simulink library "powerlib"  (Simulink 6.0)
settings: Solver=ode45  SolverMode=SingleTasking  StartTime=0.0  StopTime=10.0  RelTol=1e-3
undefined symbols (not defined in the file or in its folder): com, ctrl1, Da, DiscIntNeverNeededParam, dtha, etat, FA, find_system, Ha, j, Ka, Ki, Kv, q0, Rground, sel, st_a, st_b, st_c, sta, stb, stc, T1, T2, T3, T4
libraries: powerlib_models x30, powerlib x25, simulink_extras x6, powerlib_extras x3, simulink x2
(part 6 of 7)

== system powerlib/Machines/Excitation System ==
  note: The simulink model of the Excitation system
      | can be found in the Continuous and Discrete
      | libraries of powerlib_models.
  vref : Inport  Port=1  LatchInput=off
  vd : Inport  Port=2  LatchInput=off
  vq : Inport  Port=3  LatchInput=off
  vstab : Inport  Port=4  LatchInput=off
  Source : powerlib_models/Continuous/Excitation_System  tr=tr  reg=reg  exc=exc  tgr=tgr  damp=damp  sat=sat  lim=lim  v0=v0
  Vf : Outport  InitialOutput=0
  wires:
  Source/1 -> Vf/1
  vref/1 -> Source/1
  vd/1 -> Source/2
  vq/1 -> Source/3
  vstab/1 -> Source/4

== system powerlib/Machines/Generic Power System Stabilizer ==
  note: The simulink model of the Generic Power
      | System Stabilizer can be found in the
      | Continuous and Discrete libraries
      | of powerlib_models.
  In : Inport  Port=1  LatchInput=off
  Source : powerlib_models/Continuous/PSS  Tsensor=Tsensor  K=K  Twashout=Twashout  Tleadlag1=Tleadlag1  Tleadlag2=Tleadlag2  VSlimits=VSlimits  Vinit=Vinit  Plot_On=off  MagdB_On=on  FreqRange=logspace(-2,2,500)
  Vstab : Outport  InitialOutput=0
  wires:
  Source/1 -> Vstab/1
  In/1 -> Source/1

== system powerlib/Machines/Hydraulic Turbine and Governor ==
  note: The simulink model of the Hydraulic Turbine and
      | Governor can be found in the Continuous and
      | Discrete libraries of powerlib_models.
  wref : Inport  Port=1  LatchInput=off
  Pref : Inport  Port=2  LatchInput=off
  we : Inport  Port=3  LatchInput=off
  Pe0 : Inport  Port=4  LatchInput=off
  dw : Inport  Port=5  LatchInput=off
  Source : powerlib_models/Continuous/HTG  sm=sm  gate=gate  reg=reg  hyd=hyd  dref=dref  po=po
  Pm : Outport  InitialOutput=0
  gate : Outport  Port=2  InitialOutput=0
  wires:
  wref/1 -> Source/1
  Pref/1 -> Source/2
  we/1 -> Source/3
  Pe0/1 -> Source/4
  dw/1 -> Source/5
  Source/2 -> gate/1
  Source/1 -> Pm/1

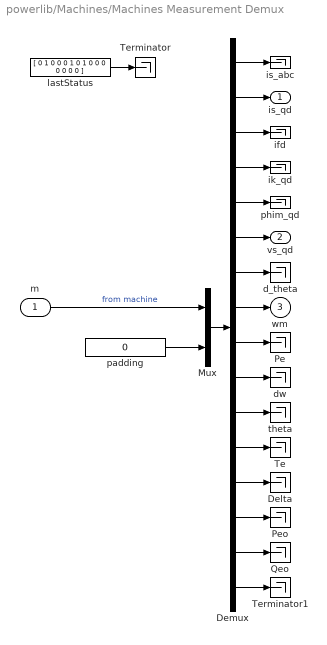
== system powerlib/Machines/Machines Measurement Demux ==
  m : Inport  Port=1  LatchInput=off
  Delta : Terminator
      settings: Tag=port13
  Demux : Demux  Outputs="[3 2 1 3 2 2 1 1 1 1 1 1 1 1 1,  1]"
  Mux : Mux  Inputs=2
  Pe : Terminator
      settings: Tag=port9
  Peo : Terminator
      settings: Tag=port14
  Qeo : Terminator
      settings: Tag=port15
  Te : Terminator
      settings: Tag=port12
  Terminator : Terminator
  Terminator1 : Terminator
  d_theta : Terminator
      settings: Tag=port7
  dw : Terminator
      settings: Tag=port10
  ifd : Terminator
      settings: Tag=port3
  ik_qd : Terminator
      settings: Tag=port4
  is_abc : Terminator
      settings: Tag=port1
  lastStatus : Constant  Value="[ 0  1  0  0  0  1  0  1  0  0  0  0  0  0  0 ]"
  padding : Constant  Value=0
  phim_qd : Terminator
      settings: Tag=port5
  theta : Terminator
      settings: Tag=port11
  is_qd : Outport  Tag=port2
  vs_qd : Outport  Tag=port6  Port=2
  wm : Outport  Tag=port8  Port=3
  wires:
  padding/1 -> Mux/2
  Demux/1 -> is_abc/1
  Demux/2 -> is_qd/1
  Demux/3 -> ifd/1
  Demux/4 -> ik_qd/1
  Demux/5 -> phim_qd/1
  Demux/6 -> vs_qd/1
  Demux/7 -> d_theta/1
  Demux/8 -> wm/1
  Demux/9 -> Pe/1
  Demux/10 -> dw/1
  Demux/11 -> theta/1
  Mux/1 -> Demux/1
  lastStatus/1 -> Terminator/1
  m/1 -> Mux/1  "from machine"
  Demux/16 -> Terminator1/1
  Demux/15 -> Qeo/1
  Demux/14 -> Peo/1
  Demux/13 -> Delta/1
  Demux/12 -> Te/1

== system powerlib/Machines/Multi-Band Power System Stabilizer ==
  note: The simulink model of the Multi-Band Power
      | System Stabilizer can be found in the
      | Continuous and Discrete libraries
      | of powerlib_models.
  dw : Inport  Port=1  LatchInput=off
  Source : powerlib_models/Continuous/MBPSS  OperationMode=Simplified settings  Kg=Kg  GL=GL  GI=GI  GH=GH  GLd=GLd  TcLF=TcLF  GId=GId  TcIF=TcIF  GHd=GHd  TcHF=TcHF  LIM=LIM  Plot_On=off  MagdB_On=off  FreqRange=logspace(-2,2,500)
  Vstab : Outport  InitialOutput=0
  wires:
  dw/1 -> Source/1
  Source/1 -> Vstab/1

== system powerlib/Machines/Permanent Magnet Synchronous Machine ==
  Tm : Inport  Orientation=left  Port=1  LatchInput=off
  ASM : PMComponent  PhysicalDomain=powersysdomain  LeftPortType=p1  RightPortType=p1  LConnTagsString=A|B  RConnTagsString=__newr0
      mask Type: InnerPowersysBlock
  Measurement list : Subsystem
  PMSM_mechanics : powerlib_models/Continuous/PMSM_mechanics  Orientation=left
  Source : powerlib_models/Continuous/PM_synchronous_machine
  A : PMIOPort  Port=1  Side=Left
  B : PMIOPort  Port=2  Side=Left
  C : PMIOPort  Orientation=left  Port=3  Side=Left
  m : Outport  InitialOutput=0
  tag scope: LibraryTag=global
  wires:
  Measurement list/1(Out1) -> m/1
  [LibraryTag] -> Source/1
  Source/1 -> [LibraryTag]
  Source/3 -> PMSM_mechanics/2
  Source/2 -> Measurement list/1(m_e)
  Tm/1 -> PMSM_mechanics/1
  PMSM_mechanics/3 -> Measurement list/2(m_m)
  PMSM_mechanics/2 -> Source/3
  PMSM_mechanics/1 -> Source/2
  connections:
  C/RConn1 -- ASM/RConn1
  B/RConn1 -- ASM/LConn2
  A/RConn1 -- ASM/LConn1

== system powerlib/Machines/Simplified Synchronous Machine SI Units ==
  Pm : Inport  Orientation=left  Port=1  LatchInput=off
  E : Inport  Port=2  LatchInput=off
  Measurement list : Subsystem
  SSM : PMComponent  PhysicalDomain=powersysdomain  LeftPortType=p1  RightPortType=p1  LConnTagsString=__newl0  RConnTagsString=A|B|C
      mask Type: InnerPowersysBlock
  SSM_mechanics : powerlib_models/Continuous/SSM_mechanics  Orientation=left
  Source : powerlib_models/Continuous/simplified_sync_mach
  A : PMIOPort  Orientation=left  Port=1  Side=Right
  B : PMIOPort  Orientation=left  Port=2  Side=Right
  C : PMIOPort  Orientation=left  Port=3  Side=Right
  m : Outport  InitialOutput=0
  tag scope: LibraryTag=global
  wires:
  Measurement list/1(Out1) -> m/1
  [LibraryTag] -> Source/1
  E/1 -> Source/2
  Source/1 -> [LibraryTag]
  Source/2 -> Measurement list/1(In1)
  Source/3 -> SSM_mechanics/2
  Pm/1 -> SSM_mechanics/1
  SSM_mechanics/1 -> Source/3
  SSM_mechanics/2 -> Source/4
  connections:
  SSM/RConn3 -- C/RConn1
  SSM/RConn1 -- A/RConn1
  SSM/RConn2 -- B/RConn1

== system powerlib/Machines/Simplified Synchronous Machine pu Units ==
  Pm : Inport  Orientation=left  Port=1  LatchInput=off
  E : Inport  Port=2  LatchInput=off
  Measurement list : Subsystem
  SSM : PMComponent  PhysicalDomain=powersysdomain  LeftPortType=p1  RightPortType=p1  LConnTagsString=__newl0  RConnTagsString=A|B|C
      mask Type: InnerPowersysBlock
  SSM_mechanics : powerlib_models/Continuous/SSM_mechanics  Orientation=left
  Source : powerlib_models/Continuous/simplified_sync_mach
  A : PMIOPort  Orientation=left  Port=1  Side=Right
  B : PMIOPort  Orientation=left  Port=2  Side=Right
  C : PMIOPort  Orientation=left  Port=3  Side=Right
  m : Outport  InitialOutput=0
  tag scope: LibraryTag=global
  wires:
  Measurement list/1(Out1) -> m/1
  [LibraryTag] -> Source/1
  Source/1 -> [LibraryTag]
  Source/2 -> Measurement list/1(In1)
  Pm/1 -> SSM_mechanics/1
  Source/3 -> SSM_mechanics/2
  E/1 -> Source/2
  SSM_mechanics/1 -> Source/3
  SSM_mechanics/2 -> Source/4
  connections:
  SSM/RConn3 -- C/RConn1
  SSM/RConn1 -- A/RConn1
  SSM/RConn2 -- B/RConn1

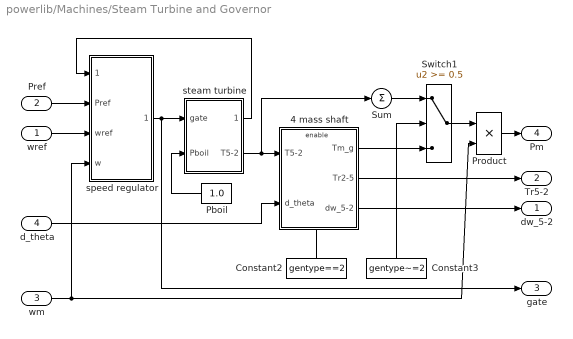
== system powerlib/Machines/Steam Turbine and Governor ==
  wref : Inport  Port=1  LatchInput=off
  Pref : Inport  Port=2  LatchInput=off
  wm : Inport  Port=3  LatchInput=off
  d_theta : Inport  Port=4  LatchInput=off
  4 mass shaft : Subsystem  TreatAsAtomicUnit=on
  Constant2 : Constant  Orientation=up  Value=gentype==2
  Constant3 : Constant  Orientation=up  Value=gentype~=2
  Pboil : Constant  Orientation=left  Value=1.0
  Product : Product  SaturateOnIntegerOverflow=on  InputSameDT=on
  Sum : Sum  Inputs=+  SaturateOnIntegerOverflow=on  InputSameDT=on
  Switch1 : Switch  Threshold=0.5  InputSameDT=on
  speed regulator : Subsystem  mask(Speed regulator for thermal turbine){Rp=reg1(2), Kp=reg1(1), Dz=reg1(3), Tsr=reg2(1), Tsm=reg2(2), lim=reg3, g0=q0}
      mask prompts: Rp "Permanent droop Rp:"; Kp "Regulator gain Kp:"; Dz "Regulator dead zone limit Dz (p.u.):"; Tsr "Speed relay time constant Tsr (s):"; Tsm "Servo motor time constant Tsv:"; lim "Gate opening limits [ vgmin,vgmax (p.u./s)  gmin,gmax (p.u.)]:"; g0 "Initial gate opening g0 (p.u.):"
      mask init:
      | vgmin=lim(1); vgmax=lim(2); gmin=lim(3); gmax=lim(4);
  steam turbine : Subsystem  mask(Thermal turbine){Fa=FA, Ta=turb1, f0=q0}
      mask prompts: Fa "Generator 1 torque fractions [ F1  F2  F3  F4 ]:"; Ta "Time constants [ T1  T2  T3  T4 ] (s):"; f0 "Initial flows f0:"
      mask init:
      | F2=Fa(1); F3=Fa(2); F4=Fa(3); F5=Fa(4);
      | if Ta(1)==0, T1=1; else T1=Ta(1); end; if Ta(2)==0, T2=1; else T2=Ta(2); end
      | if Ta(3)==0, T3=1; else T3=Ta(3); end; if Ta(4)==0, T4=1; else T4=Ta(4); end
  dw_5-2 : Outport
  Tr5-2 : Outport  Port=2
  gate : Outport  Port=3
  Pm : Outport  Port=4
  wires:
  wm/1 -> Product/2, speed regulator/4(w)
  Pref/1 -> speed regulator/2(Pref)
  wref/1 -> speed regulator/3(wref)
  Pboil/1 -> steam turbine/2(Pboil)
  Product/1 -> Pm/1
  4 mass shaft/2(Tr2-5) -> Tr5-2/1
  Switch1/1 -> Product/1
  4 mass shaft/1(Tm_g) -> Switch1/3
  Sum/1 -> Switch1/1
  Constant3/1 -> Switch1/2
  d_theta/1 -> 4 mass shaft/2(d_theta)
  steam turbine/1(flowHp) -> speed regulator/1(flowHP)
  steam turbine/2(T5-2) -> 4 mass shaft/1(T5-2), Sum/1
  4 mass shaft/3(dw_5-2) -> dw_5-2/1
  speed regulator/1(gate opening) -> steam turbine/1(gate), gate/1
  Constant2/1 -> 4 mass shaft/Enable

== system powerlib/Machines/Synchronous Machine SI Fundamental ==
  Pm : Inport  Orientation=left  Port=1  LatchInput=off
  Vf_ : Inport  Port=2  LatchInput=off
  Measurement list : Subsystem
  SM : PMComponent  PhysicalDomain=powersysdomain  LeftPortType=p1  RightPortType=p1  LConnTagsString=__newl0  RConnTagsString=B|C
      mask Type: InnerPowersysBlock
  SM_mechanics : powerlib_models/Continuous/SM_mechanics  Orientation=left
  Source : powerlib_models/Continuous/synchronous_machine
  A : PMIOPort  Port=1  Side=Right
  B : PMIOPort  Orientation=left  Port=2  Side=Right
  C : PMIOPort  Orientation=left  Port=3  Side=Right
  m : Outport  InitialOutput=0
  tag scope: LibraryTag=global
  wires:
  Source/1 -> [LibraryTag]
  [LibraryTag] -> Source/1
  Source/3 -> SM_mechanics/1
  Vf_/1 -> Source/2
  Measurement list/1(m) -> m/1
  SM_mechanics/1 -> Measurement list/2(m_m)
  Source/2 -> Measurement list/1(m_e)
  SM_mechanics/2 -> Source/3
  SM_mechanics/3 -> Source/4
  Pm/1 -> SM_mechanics/2
  connections:
  SM/RConn2 -- C/RConn1
  SM/LConn1 -- A/RConn1
  SM/RConn1 -- B/RConn1

== system powerlib/Machines/Synchronous Machine pu Fundamental ==
  Pm : Inport  Orientation=left  Port=1  LatchInput=off
  Vf_ : Inport  Port=2  LatchInput=off
  Measurement list : Subsystem
  SM : PMComponent  PhysicalDomain=powersysdomain  LeftPortType=p1  RightPortType=p1  LConnTagsString=__newl0  RConnTagsString=B|C
      mask Type: InnerPowersysBlock
  SM_mechanics : powerlib_models/Continuous/SM_mechanics  Orientation=left
  Source : powerlib_models/Continuous/synchronous_machine
  A : PMIOPort  Port=1  Side=Right
  B : PMIOPort  Orientation=left  Port=2  Side=Right
  C : PMIOPort  Orientation=left  Port=3  Side=Right
  m : Outport  InitialOutput=0
  tag scope: LibraryTag=global
  wires:
  Measurement list/1(m) -> m/1
  Source/1 -> [LibraryTag]
  [LibraryTag] -> Source/1
  Vf_/1 -> Source/2
  Pm/1 -> SM_mechanics/2
  Source/3 -> SM_mechanics/1
  Source/2 -> Measurement list/1(m_e)
  SM_mechanics/1 -> Measurement list/2(m_m)
  SM_mechanics/2 -> Source/3
  SM_mechanics/3 -> Source/4
  connections:
  C/RConn1 -- SM/RConn2
  B/RConn1 -- SM/RConn1
  A/RConn1 -- SM/LConn1

== system powerlib/Machines/Synchronous Machine pu Standard ==
  Pm : Inport  Orientation=left  Port=1  LatchInput=off
  Vf_ : Inport  Port=2  LatchInput=off
  Measurement list : Subsystem
  SM : PMComponent  PhysicalDomain=powersysdomain  LeftPortType=p1  RightPortType=p1  LConnTagsString=__newl0  RConnTagsString=B|C
      mask Type: InnerPowersysBlock
  SM_mechanics : powerlib_models/Continuous/SM_mechanics  Orientation=left
  Source : powerlib_models/Continuous/synchronous_machine
  A : PMIOPort  Port=1  Side=Right
  B : PMIOPort  Orientation=left  Port=2  Side=Right
  C : PMIOPort  Orientation=left  Port=3  Side=Right
  m : Outport  InitialOutput=0
  tag scope: LibraryTag=global
  wires:
  Source/1 -> [LibraryTag]
  [LibraryTag] -> Source/1
  Source/3 -> SM_mechanics/1
  Vf_/1 -> Source/2
  Source/2 -> Measurement list/1(m_e)
  SM_mechanics/1 -> Measurement list/2(m_m)
  Measurement list/1(m) -> m/1
  SM_mechanics/2 -> Source/3
  SM_mechanics/3 -> Source/4
  Pm/1 -> SM_mechanics/2
  connections:
  A/RConn1 -- SM/LConn1
  SM/RConn2 -- C/RConn1
  SM/RConn1 -- B/RConn1

== system powerlib/Measurements/  Extra Library  ==

== system powerlib/Measurements/  Extra Library 1 ==

== system powerlib/Measurements/  Extra Library 2 ==

== system powerlib/Measurements/Current Measurement ==
  CurrentMeasurement : PMComponent  PhysicalDomain=powersysdomain  LeftPortType=p1  RightPortType=p1  LConnTagsString=a  RConnTagsString=__new0
      mask Type: InnerPowersysBlock
  model : powerlib_models/Continuous/Measurement
  + : PMIOPort  Port=1  Side=Left
  - : PMIOPort  Orientation=left  Port=2  Side=Right
  i : Outport  InitialOutput=0
  wires:
  [LibraryTag] -> model/1
  model/1 -> i/1
  connections:
  -/RConn1 -- CurrentMeasurement/RConn1
  +/RConn1 -- CurrentMeasurement/LConn1

== system powerlib/Measurements/Multimeter ==
  Gain2 : Gain  Gain=Gain  SaturateOnIntegerOverflow=on
  Mode : Constant  Value=Display
  Selector : Selector  Elements=SelectionMode  InputPortWidth=SignalLength
  StoreData : Subsystem  Orientation=down  TreatAsAtomicUnit=on  mask{RowMax=inf}
      mask prompts: RowMax "Maximum Number of rows"
      mask init:
      | powericon('psbloadfunction',gcb,'StoreDataBlock','Initialize');
      settings: CopyFcn=powericon('psbloadfunction',gcb,'StoreDataBlock','UpdateVariableName');
  model : powerlib_models/Continuous/Measurement
  selection : Selector  Elements=sel  InputPortWidth=L
  Out1 : Outport
  wires:
  Mode/1 -> StoreData/Enable
  selection/1 -> Gain2/1
  [gotomultimeterPSB] -> selection/1
  Gain2/1 -> model/1
  model/1 -> Selector/1
  Selector/1 -> Out1/1, StoreData/1(In1)

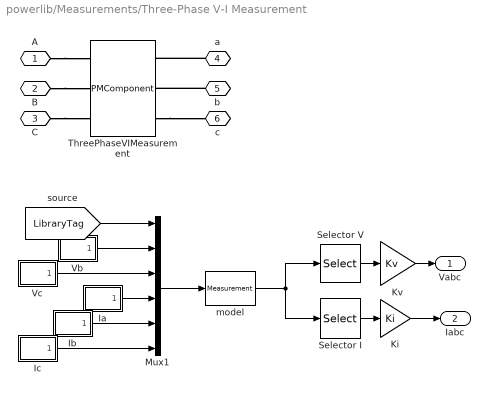
== system powerlib/Measurements/Three-Phase V-I Measurement ==
  Ia : Subsystem
  Ib : Subsystem
  Ic : Subsystem
  Ki : Gain  Gain=Ki  SaturateOnIntegerOverflow=on
  Kv : Gain  Gain=Kv  SaturateOnIntegerOverflow=on
  Mux1 : Mux  Inputs=6
  Selector I : Selector  Elements=SelectionModeI  InputPortWidth=SignalLength
  Selector V : Selector  Elements=SelectionModeV  InputPortWidth=SignalLength
  ThreePhaseVIMeasurement : PMComponent  PhysicalDomain=powersysdomain  LeftPortType=p1  RightPortType=p1  LConnTagsString=A|B|C  RConnTagsString=a|b|c
      mask Type: InnerPowersysBlock
  Vb : Subsystem
  Vc : Subsystem
  model : powerlib_models/Continuous/Measurement
  A : PMIOPort  Port=1  Side=Left
  B : PMIOPort  Port=2  Side=Left
  C : PMIOPort  Port=3  Side=Left
  a : PMIOPort  Orientation=left  Port=4  Side=Right
  b : PMIOPort  Orientation=left  Port=5  Side=Right
  c : PMIOPort  Orientation=left  Port=6  Side=Right
  Vabc : Outport
  Iabc : Outport  Port=2
  wires:
  Vb/1(Out1) -> Mux1/2
  Vc/1(Out1) -> Mux1/3
  Ia/1(Out1) -> Mux1/4
  Ib/1(Out1) -> Mux1/5
  Ic/1(Out1) -> Mux1/6
  [LibraryTag] -> Mux1/1
  Selector I/1 -> Ki/1
  Selector V/1 -> Kv/1
  Ki/1 -> Iabc/1
  Kv/1 -> Vabc/1
  Mux1/1 -> model/1
  model/1 -> Selector V/1, Selector I/1
  connections:
  B/RConn1 -- ThreePhaseVIMeasurement/LConn2
  A/RConn1 -- ThreePhaseVIMeasurement/LConn1
  C/RConn1 -- ThreePhaseVIMeasurement/LConn3
  ThreePhaseVIMeasurement/RConn3 -- c/RConn1
  b/RConn1 -- ThreePhaseVIMeasurement/RConn2
  a/RConn1 -- ThreePhaseVIMeasurement/RConn1

== system powerlib/Measurements/Voltage Measurement ==
  VoltageMeasurement : PMComponent  PhysicalDomain=powersysdomain  LeftPortType=p1  RightPortType=p1  LConnTagsString=+  RConnTagsString=-
      mask Type: InnerPowersysBlock
  model : powerlib_models/Continuous/Measurement
  + : PMIOPort  Port=1  Side=Left
  - : PMIOPort  Orientation=left  Port=2  Side=Left
  v : Outport  InitialOutput=0
  wires:
  [LibraryTag] -> model/1
  model/1 -> v/1
  connections:
  +/RConn1 -- VoltageMeasurement/LConn1
  -/RConn1 -- VoltageMeasurement/RConn1

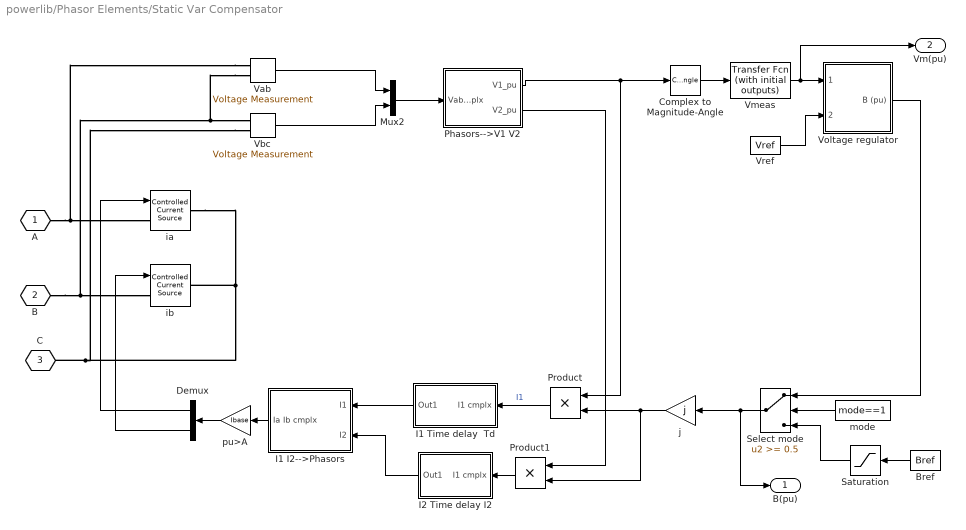
== system powerlib/Phasor Elements/Static Var Compensator ==
  Bref : Constant  Orientation=left  Value=Bref
  Complex to Magnitude-Angle : ComplexToMagnitudeAngle  Output=Magnitude
  Demux : Demux  Orientation=left  Outputs=2
  I1 I2-->Phasors : Subsystem  Orientation=left
  I1 Time delay  Td : Subsystem  Orientation=left
  I2 Time delay I2 : Subsystem  Orientation=left
  Mux2 : Mux  Inputs=2
  Phasors-->V1 V2 : Subsystem
  Product : Product  Orientation=left  SaturateOnIntegerOverflow=on  InputSameDT=on
  Product1 : Product  Orientation=left  SaturateOnIntegerOverflow=on  InputSameDT=on
  Saturation : Saturate  Orientation=left  UpperLimit=Bmax  LowerLimit=Bmin
  Select mode : Switch  Orientation=left  Threshold=0.5  InputSameDT=on
  Vab : powerlib/Measurements/Voltage Measurement  PhasorSimulation=off  OutputType=Complex  PSBequivalent=0
  Vbc : powerlib/Measurements/Voltage Measurement  PhasorSimulation=off  OutputType=Complex  PSBequivalent=0
  Vmeas : simulink_extras/Additional Linear/Transfer Fcn (with initial outputs)  N=[1]  D="[Tm  1]"  Y0=Vref  U0=Vref
  Voltage regulator : Subsystem
  Vref : Constant  Value=Vref
  ia : powerlib/Electrical Sources/Controlled Current Source  Description=source block  Initialize=off  Amplitude=0  Phase=0  Frequency=0  Measurements=None
  ib : powerlib/Electrical Sources/Controlled Current Source  Description=source block  Initialize=off  Amplitude=0  Phase=0  Frequency=0  Measurements=None
  j : Gain  Orientation=left  Gain=j  SaturateOnIntegerOverflow=on
  mode : Constant  Orientation=left  Value=mode==1
  pu>A : Gain  Orientation=left  Gain=Ibase  SaturateOnIntegerOverflow=on
  A : PMIOPort  Port=1  Side=Left
  B : PMIOPort  Port=2  Side=Left
  C : PMIOPort  Port=3  Side=Left
  B(pu) : Outport
  Vm(pu) : Outport  Port=2
  wires:
  Saturation/1 -> Select mode/3
  Demux/2 -> ib/1
  Demux/1 -> ia/1
  mode/1 -> Select mode/2
  Voltage regulator/1(B (pu)) -> Select mode/1
  Bref/1 -> Saturation/1
  Select mode/1 -> B(pu)/1, j/1
  Mux2/1 -> Phasors-->V1 V2/1(Vab Vbc cmplx)
  Phasors-->V1 V2/1(V1_pu) -> Complex to Magnitude-Angle/1, Product/1
  Vref/1 -> Voltage regulator/2(Vref (pu))
  Vmeas/1 -> Voltage regulator/1(V1meas (pu)), Vm(pu)/1
  I1 I2-->Phasors/1(Ia Ib cmplx) -> pu>A/1
  I2 Time delay I2/1(Out1) -> I1 I2-->Phasors/2(I2)
  Complex to Magnitude-Angle/1 -> Vmeas/1
  Vab/1 -> Mux2/1
  Vbc/1 -> Mux2/2
  I1 Time delay  Td/1(Out1) -> I1 I2-->Phasors/1(I1)
  pu>A/1 -> Demux/1
  Product/1 -> I1 Time delay  Td/1(I1 cmplx)  "I1"
  j/1 -> Product/2, Product1/2
  Phasors-->V1 V2/2(V2_pu) -> Product1/1
  Product1/1 -> I2 Time delay I2/1(I1 cmplx)
  connections:
  Vbc/LConn2 -- C/RConn1 -- ib/RConn1 -- ia/RConn1
  Vab/LConn2 -- Vbc/LConn1 -- ib/LConn1 -- B/RConn1
  Vab/LConn1 -- ia/LConn1 -- A/RConn1

== system powerlib/Power Electronics/  Extra Library  ==

== system powerlib/Power Electronics/  Extra Library 1 ==

== system powerlib/Power Electronics/Detailed Thyristor ==
  g : Inport  Port=1  LatchInput=off
  DetailedThyristor : PMComponent  PhysicalDomain=powersysdomain  LeftPortType=p1  RightPortType=p1  LConnTagsString=a  RConnTagsString=__new0
      mask Type: InnerPowersysBlock
  Measurement list : Subsystem
  a : PMIOPort  Port=1  Side=Left
  k : PMIOPort  Orientation=left  Port=2  Side=Right
  m : Outport  InitialOutput=0
  tag scope: LibraryTag=global
  wires:
  g/1 -> [LibraryTag]
  [LibraryTag] -> Measurement list/1(In1)
  Measurement list/1(Out1) -> m/1
  connections:
  DetailedThyristor/RConn1 -- k/RConn1
  a/RConn1 -- DetailedThyristor/LConn1

== system powerlib/Power Electronics/Diode ==
  Diode : PMComponent  PhysicalDomain=powersysdomain  LeftPortType=p1  RightPortType=p1  LConnTagsString=a  RConnTagsString=__new0
      mask Type: InnerPowersysBlock
  Measurement list : Subsystem
  m : Terminator
  a : PMIOPort  Port=1  Side=Left
  k : PMIOPort  Orientation=left  Port=2  Side=Right
  wires:
  [LibraryTag] -> Measurement list/1(In1)
  Measurement list/1(Out1) -> m/1
  connections:
  Diode/RConn1 -- k/RConn1
  a/RConn1 -- Diode/LConn1

== system powerlib/Power Electronics/Gto ==
  g : Inport  Port=1  LatchInput=off
  GTO : PMComponent  PhysicalDomain=powersysdomain  LeftPortType=p1  RightPortType=p1  LConnTagsString=a  RConnTagsString=__new0
      mask Type: InnerPowersysBlock
  Measurement list : Subsystem
  a : PMIOPort  Port=1  Side=Left
  k : PMIOPort  Orientation=left  Port=2  Side=Right
  m : Outport  InitialOutput=0
  tag scope: LibraryTag=global
  wires:
  g/1 -> [LibraryTag]
  [LibraryTag] -> Measurement list/1(In1)
  Measurement list/1(Out1) -> m/1
  connections:
  GTO/RConn1 -- k/RConn1
  a/RConn1 -- GTO/LConn1

== system powerlib/Power Electronics/IGBT ==
  g : Inport  Port=1  LatchInput=off
  IGBT : PMComponent  PhysicalDomain=powersysdomain  LeftPortType=p1  RightPortType=p1  LConnTagsString=a  RConnTagsString=__new0
      mask Type: InnerPowersysBlock
  Measurement list : Subsystem
  C : PMIOPort  Port=1  Side=Left
  E : PMIOPort  Orientation=left  Port=2  Side=Right
  m : Outport
  tag scope: LibraryTag=global
  wires:
  [LibraryTag] -> Measurement list/1(In1)
  g/1 -> [LibraryTag]
  Measurement list/1(Out1) -> m/1
  connections:
  IGBT/RConn1 -- E/RConn1
  C/RConn1 -- IGBT/LConn1

== system powerlib/Power Electronics/Ideal Switch ==
  g : Inport  Port=1  LatchInput=off
  IdealSwitch : PMComponent  PhysicalDomain=powersysdomain  LeftPortType=p1  RightPortType=p1  LConnTagsString=a  RConnTagsString=__new0
      mask Type: InnerPowersysBlock
  Measurement list : Subsystem
  1 : PMIOPort  Port=1  Side=Left
  2 : PMIOPort  Orientation=left  Port=2  Side=Right
  m : Outport
  tag scope: LibraryTag=global
  wires:
  [LibraryTag] -> Measurement list/1(In1)
  g/1 -> [LibraryTag]
  Measurement list/1(Out1) -> m/1
  connections:
  IdealSwitch/RConn1 -- 2/RConn1
  1/RConn1 -- IdealSwitch/LConn1

== system powerlib/Power Electronics/Mosfet ==
  g : Inport  Port=1  LatchInput=off
  Measurement list : Subsystem
  Mosfet : PMComponent  PhysicalDomain=powersysdomain  LeftPortType=p1  RightPortType=p1  LConnTagsString=a  RConnTagsString=__new0
      mask Type: InnerPowersysBlock
  d : PMIOPort  Port=1  Side=Left
  s : PMIOPort  Orientation=left  Port=2  Side=Right
  m : Outport
  tag scope: LibraryTag=global
  wires:
  g/1 -> [LibraryTag]
  [LibraryTag] -> Measurement list/1(In1)
  Measurement list/1(Out1) -> m/1
  connections:
  Mosfet/RConn1 -- s/RConn1
  d/RConn1 -- Mosfet/LConn1

== system powerlib/Power Electronics/Three-Level Bridge ==
  g : Inport  Port=1  PortDimensions=4*Arms  LatchInput=off
  Logical Operator : Logic  OutDataTypeMode=Specify via dialog  LogicDataType=float('double')
  UniversalBridge : PMComponent  PhysicalDomain=powersysdomain  LeftPortType=p1  RightPortType=p1  LConnTagsString=A|B|C  RConnTagsString=+|N|-
      mask Type: InnerPowersysBlock
  s1 : Selector  Elements=selection1  InputPortWidth=4*Arms
  s2 : Selector  Elements=selection2  InputPortWidth=4*Arms
  A : PMIOPort  Port=1  Side=Left
  B : PMIOPort  Port=2  Side=Left
  C : PMIOPort  Port=3  Side=Left
  + : PMIOPort  Orientation=left  Port=4  Side=Right
  N : PMIOPort  Orientation=left  Port=5  Side=Right
  - : PMIOPort  Orientation=left  Port=6  Side=Right
  tag scope: LibraryTag=global
  wires:
  g/1 -> s2/1, s1/1
  s2/1 -> Logical Operator/2
  s1/1 -> Logical Operator/1
  Logical Operator/1 -> [LibraryTag]
  connections:
  -/RConn1 -- UniversalBridge/RConn3
  UniversalBridge/RConn2 -- N/RConn1
  A/RConn1 -- UniversalBridge/LConn1
  B/RConn1 -- UniversalBridge/LConn2
  C/RConn1 -- UniversalBridge/LConn3
  UniversalBridge/RConn1 -- +/RConn1

== system powerlib/Power Electronics/Thyristor ==
  g : Inport  Port=1  LatchInput=off
  Measurement list : Subsystem
  Thyristor : PMComponent  PhysicalDomain=powersysdomain  LeftPortType=p1  RightPortType=p1  LConnTagsString=a  RConnTagsString=__new0
      mask Type: InnerPowersysBlock
  a : PMIOPort  Port=1  Side=Left
  k : PMIOPort  Orientation=left  Port=2  Side=Right
  m : Outport  InitialOutput=0
  tag scope: LibraryTag=global
  wires:
  g/1 -> [LibraryTag]
  [LibraryTag] -> Measurement list/1(In1)
  Measurement list/1(Out1) -> m/1
  connections:
  Thyristor/RConn1 -- k/RConn1
  a/RConn1 -- Thyristor/LConn1

== system powerlib/Power Electronics/Universal Bridge ==
  g : Inport  Port=1  LatchInput=off
  UniversalBridge : PMComponent  PhysicalDomain=powersysdomain  LeftPortType=p1  RightPortType=p1  LConnTagsString=A|B|C  RConnTagsString=+|-
      mask Type: InnerPowersysBlock
  A : PMIOPort  Port=1  Side=Left
  B : PMIOPort  Port=2  Side=Left
  C : PMIOPort  Port=3  Side=Left
  + : PMIOPort  Orientation=left  Port=4  Side=Right
  - : PMIOPort  Orientation=left  Port=5  Side=Right
  tag scope: LibraryTag=global
  wires:
  g/1 -> [LibraryTag]
  connections:
  UniversalBridge/RConn2 -- -/RConn1
  UniversalBridge/RConn1 -- +/RConn1
  A/RConn1 -- UniversalBridge/LConn1
  UniversalBridge/LConn2 -- B/RConn1
  UniversalBridge/LConn3 -- C/RConn1

== system powerlib/powergui/Subsystem ==

== system powerlib/Elements/Three-Phase Dynamic Load/Measurement list ==
  In1 : Inport  Port=1  LatchInput=off
  Bus Creator1 : BusCreator  DialogController=Simulink.DDGSource_Bus  Inputs=3
  Demux : Demux  Outputs=[1,1,1]
  Out1 : Outport
  wires:
  In1/1 -> Demux/1
  Bus Creator1/1 -> Out1/1
  Demux/2 -> Bus Creator1/2  "Active power P (W)"
  Demux/1 -> Bus Creator1/1  "Positive-sequence voltage V (pu)"
  Demux/3 -> Bus Creator1/3  "Reactive power Q (var)"

== system powerlib/Machines/Asynchronous Machine SI Units/Measurement list ==
  m_e : Inport  Port=1  LatchInput=off
  m_m : Inport  Port=2  LatchInput=off
  Bus Creator1 : BusCreator  DialogController=Simulink.DDGSource_Bus  Inputs=3
  Bus Creator2 : BusCreator  DialogController=Simulink.DDGSource_Bus  Inputs=9
  Bus Creator3 : BusCreator  DialogController=Simulink.DDGSource_Bus  Inputs=3
  Bus Creator4 : BusCreator  DialogController=Simulink.DDGSource_Bus  Inputs=9
  Demux : Demux  Outputs=[1,1,1,1,1,1,1,1,1,1,1,1,1,1,1,1,1,1]
  Demux1 : Demux  Outputs=[1,1,1]
  Out1 : Outport
  wires:
  Bus Creator3/1 -> Bus Creator1/3  "Mechanical"
  Demux/18 -> Bus Creator4/9  "Stator voltage vs_d (V)"
  Demux/17 -> Bus Creator4/8  "Stator voltage vs_q (V)"
  Demux/16 -> Bus Creator4/7  "Stator flux phis_d (V s)"
  Demux/15 -> Bus Creator4/6  "Stator flux phis_q (V s)"
  Demux1/1 -> Bus Creator3/1  "Rotor speed (wm)"
  Demux1/2 -> Bus Creator3/2  "Electromagnetic torque Te (N*m)"
  Demux1/3 -> Bus Creator3/3  "Rotor angle thetam (rad)"
  Bus Creator4/1 -> Bus Creator1/2  "Stator measurements"
  Demux/14 -> Bus Creator4/5  "Stator current is_d (A)"
  Demux/13 -> Bus Creator4/4  "Stator current  is_q (A)"
  Demux/12 -> Bus Creator4/3  "Stator current is_c (A)"
  Demux/11 -> Bus Creator4/2  "Stator current is_b (A)"
  Demux/10 -> Bus Creator4/1  "Stator current is_a (A)"
  Demux/9 -> Bus Creator2/9  "Rotor voltage Vr_d (V)"
  Demux/8 -> Bus Creator2/8  "Rotor voltage Vr_q (V)"
  Demux/7 -> Bus Creator2/7  "Rotor flux phir_d (V s)"
  Demux/6 -> Bus Creator2/6  "Rotor flux phir_q (V s)"
  Demux/5 -> Bus Creator2/5  "Rotor current  id (A)"
  Demux/4 -> Bus Creator2/4  "Rotor current  iq (A)"
  Bus Creator2/1 -> Bus Creator1/1  "Rotor measurements"
  Demux/3 -> Bus Creator2/3  "Rotor current ir_c (A)"
  Demux/2 -> Bus Creator2/2  "Rotor current ir_b (A)"
  Demux/1 -> Bus Creator2/1  "Rotor current ir_a (A)"
  Bus Creator1/1 -> Out1/1
  m_e/1 -> Demux/1
  m_m/1 -> Demux1/1

== system powerlib/Machines/Asynchronous Machine pu Units/Measurement list ==
  m_e : Inport  Port=1  LatchInput=off
  m_m : Inport  Port=2  LatchInput=off
  Bus Creator1 : BusCreator  DialogController=Simulink.DDGSource_Bus  Inputs=3
  Bus Creator2 : BusCreator  DialogController=Simulink.DDGSource_Bus  Inputs=9
  Bus Creator3 : BusCreator  DialogController=Simulink.DDGSource_Bus  Inputs=3
  Bus Creator4 : BusCreator  DialogController=Simulink.DDGSource_Bus  Inputs=9
  Demux : Demux  Outputs=[1,1,1,1,1,1,1,1,1,1,1,1,1,1,1,1,1,1]
  Demux1 : Demux  Outputs=[1,1,1]
  Out1 : Outport
  wires:
  m_e/1 -> Demux/1
  Bus Creator1/1 -> Out1/1
  Demux/1 -> Bus Creator2/1  "Rotor current ir_a (pu)"
  Demux/2 -> Bus Creator2/2  "Rotor current ir_b (pu)"
  Demux/3 -> Bus Creator2/3  "Rotor current ir_c (pu)"
  Bus Creator2/1 -> Bus Creator1/1  "Rotor measurements"
  Demux/4 -> Bus Creator2/4  "Rotor current  iq (pu)"
  Demux/5 -> Bus Creator2/5  "Rotor current  id (pu)"
  Demux/6 -> Bus Creator2/6  "Rotor flux phir_q (pu)"
  Demux/7 -> Bus Creator2/7  "Rotor flux phir_d (pu)"
  Demux/8 -> Bus Creator2/8  "Rotor voltage Vr_q (pu)"
  Demux/9 -> Bus Creator2/9  "Rotor voltage Vr_d (pu)"
  Demux/10 -> Bus Creator4/1  "Stator current is_a (pu)"
  Demux/11 -> Bus Creator4/2  "Stator current is_b (pu)"
  Demux/12 -> Bus Creator4/3  "Stator current is_c (pu)"
  Demux/13 -> Bus Creator4/4  "Stator current is_q (pu)"
  Demux/14 -> Bus Creator4/5  "Stator current is_d (pu)"
  Bus Creator4/1 -> Bus Creator1/2  "Stator measurements"
  Demux/15 -> Bus Creator4/6  "Stator flux phis_q (pu)"
  Demux/16 -> Bus Creator4/7  "Stator flux phis_d (pu)"
  Demux/17 -> Bus Creator4/8  "Stator voltage vs_q (pu)"
  Demux/18 -> Bus Creator4/9  "Stator voltage vs_d (pu)"
  Bus Creator3/1 -> Bus Creator1/3  "Mechanical"
  Demux1/1 -> Bus Creator3/1  "Rotor speed (wm)"
  Demux1/2 -> Bus Creator3/2  "Electromagnetic torque Te (pu)"
  Demux1/3 -> Bus Creator3/3  "Rotor angle thetam (rad)"
  m_m/1 -> Demux1/1

== system powerlib/Machines/DC Machine/Measurement list ==
  In1 : Inport  Port=1  LatchInput=off
  Bus Creator1 : BusCreator  DialogController=Simulink.DDGSource_Bus
  Demux : Demux  Outputs=[1,1,1,1]
  Out1 : Outport
  wires:
  In1/1 -> Demux/1
  Bus Creator1/1 -> Out1/1
  Demux/1 -> Bus Creator1/1  "Speed wm (rad/s)"
  Demux/2 -> Bus Creator1/2  "Armature current ia (A)"
  Demux/3 -> Bus Creator1/3  "Field current if (A)"
  Demux/4 -> Bus Creator1/4  "Electrical torque Te (n m)"

== system powerlib/Machines/DC Machine/Mechanics ==
  TL : Inport  Port=1  LatchInput=off
  ia : Inport  Port=2  LatchInput=off
  if : Inport  Port=3  LatchInput=off
  Coulomb (Tf) & Viscous ( Bm*w)  Friction Torques : simulink/Discontinuities/Coulomb & Viscous Friction  Orientation=left  offset=Tf  gain=Bm
  Gain2 : Gain  Gain=1/J  SaturateOnIntegerOverflow=on
  Integrator : Integrator  InitialCondition=w0  ZeroCross=off
  Mux : Mux
  Product : Product  SaturateOnIntegerOverflow=on  InputSameDT=on
  Product1 : Product  SaturateOnIntegerOverflow=on  InputSameDT=on
  Sum : Sum  Inputs=-+-  SaturateOnIntegerOverflow=on  InputSameDT=on
  Transfer Fcn2 : TransferFcn  Numerator=[Laf]  Denominator=[20e-6 1]
  FCEM : Outport
  m : Outport  Port=2
  wires:
  Coulomb (Tf) & Viscous ( Bm*w)  Friction Torques/1 -> Sum/3
  Transfer Fcn2/1 -> Product/2, Product1/2
  Product1/1 -> Mux/4, Sum/2  "Te"
  Integrator/1 -> Product/1, Mux/1, Coulomb (Tf) & Viscous ( Bm*w)  Friction Torques/1  "w"
  Gain2/1 -> Integrator/1
  Sum/1 -> Gain2/1
  TL/1 -> Sum/1
  if/1 -> Transfer Fcn2/1, Mux/3  "If"
  ia/1 -> Product1/1, Mux/2  "ia"
  Product/1 -> FCEM/1  "E fcem"
  Mux/1 -> m/1

== system powerlib/Machines/Discrete DC Machine/Measurement list ==
  In1 : Inport  Port=1  LatchInput=off
  Bus Creator1 : BusCreator  DialogController=Simulink.DDGSource_Bus
  Demux : Demux  Outputs=[1,1,1,1]
  Out1 : Outport
  wires:
  Demux/4 -> Bus Creator1/4  "Electrical torque Te (n m)"
  Demux/3 -> Bus Creator1/3  "Field current if (A)"
  Demux/2 -> Bus Creator1/2  "Armature current ia (A)"
  Demux/1 -> Bus Creator1/1  "Speed wm (rad/s)"
  Bus Creator1/1 -> Out1/1
  In1/1 -> Demux/1

== system powerlib/Machines/Discrete DC Machine/Mechanics ==
  TL : Inport  Port=1  LatchInput=off
  iA : Inport  Port=2  LatchInput=off
  iF : Inport  Port=3  LatchInput=off
  Coulomb (Tf) & Viscous ( Bm*w)  Friction Torques : simulink/Discontinuities/Coulomb & Viscous Friction  Orientation=left  offset=Tf  gain=Bm
  Discrete-Time Integrator : DiscreteIntegrator  InitialCondition=w0  SampleTime=Ts  SaturateOnIntegerOverflow=on  ICPrevOutput=DiscIntNeverNeededParam  ICPrevScaledInput=DiscIntNeverNeededParam
  Gain2 : Gain  Gain=1/J  SaturateOnIntegerOverflow=on
  Gain3 : Gain  Gain=Laf  SaturateOnIntegerOverflow=on
  Mux : Mux
  Product : Product  Orientation=left  SaturateOnIntegerOverflow=on  InputSameDT=on
  Product1 : Product  SaturateOnIntegerOverflow=on  InputSameDT=on
  Sum : Sum  Inputs=-+-  SaturateOnIntegerOverflow=on  InputSameDT=on
  Unit Delay : UnitDelay  SampleTime=Ts
  m : Outport
  FCEM : Outport  Orientation=left  Port=2
  wires:
  Product/1 -> FCEM/1
  Mux/1 -> m/1
  Unit Delay/1 -> Product1/2, Product/2
  Gain3/1 -> Unit Delay/1
  iA/1 -> Mux/2, Product1/1  "Ia"
  iF/1 -> Mux/3, Gain3/1  "If"
  TL/1 -> Sum/1
  Sum/1 -> Gain2/1
  Gain2/1 -> Discrete-Time Integrator/1
  Discrete-Time Integrator/1 -> Coulomb (Tf) & Viscous ( Bm*w)  Friction Torques/1, Product/1, Mux/1  "w"
  Product1/1 -> Sum/2, Mux/4  "Te"
  Coulomb (Tf) & Viscous ( Bm*w)  Friction Torques/1 -> Sum/3

== system powerlib/Machines/Permanent Magnet Synchronous Machine/Measurement list ==
  m_e : Inport  Port=1  LatchInput=off
  m_m : Inport  Port=2  LatchInput=off
  Bus Creator1 : BusCreator  DialogController=Simulink.DDGSource_Bus  Inputs=10
  Demux : Demux  Outputs=[1,1,1,1,1,1,1]
  Demux1 : Demux  Outputs=[1,1,1]
  Out1 : Outport
  wires:
  m_e/1 -> Demux/1
  Bus Creator1/1 -> Out1/1
  Demux/1 -> Bus Creator1/1  "Stator current is_a (A)"
  Demux/2 -> Bus Creator1/2  "Stator current is_b (A)"
  Demux/3 -> Bus Creator1/3  "Stator current is_c (A)"
  Demux/4 -> Bus Creator1/4  "Stator current is_q (A)"
  Demux/5 -> Bus Creator1/5  "Stator current is_d (A)"
  Demux/6 -> Bus Creator1/6  "Stator voltage Vs_q (V)"
  Demux/7 -> Bus Creator1/7  "Stator voltage Vs_d (V)"
  Demux1/1 -> Bus Creator1/8  "Rotor speed wm (rad/s)"
  Demux1/2 -> Bus Creator1/9  "Rotor angle thetam (rad)"
  Demux1/3 -> Bus Creator1/10  "Electromagnetic torque Te (N*m)"
  m_m/1 -> Demux1/1

== system powerlib/Machines/Simplified Synchronous Machine SI Units/Measurement list ==
  In1 : Inport  Port=1  LatchInput=off
  Bus Creator1 : BusCreator  DialogController=Simulink.DDGSource_Bus  Inputs=12
  Demux : Demux  Outputs=[1,1,1,1,1,1,1,1,1,1,1,1]
  Out1 : Outport
  wires:
  In1/1 -> Demux/1
  Bus Creator1/1 -> Out1/1
  Demux/1 -> Bus Creator1/1  "Stator current is_a (A)"
  Demux/2 -> Bus Creator1/2  "Stator current is_b (A)"
  Demux/3 -> Bus Creator1/3  "Stator current is_c (A)"
  Demux/4 -> Bus Creator1/4  "Terminal voltage Va (V)"
  Demux/5 -> Bus Creator1/5  "Terminal voltage Vb (V)"
  Demux/6 -> Bus Creator1/6  "Terminal voltage Vc (V)"
  Demux/7 -> Bus Creator1/7  "Internal voltage Ea (V)"
  Demux/8 -> Bus Creator1/8  "Internal voltage Eb (V)"
  Demux/9 -> Bus Creator1/9  "Internal voltage Ec (V)"
  Demux/10 -> Bus Creator1/10  "Rotor angle theta (rad)"
  Demux/11 -> Bus Creator1/11  "Rotor speed wm (rad/s)"
  Demux/12 -> Bus Creator1/12  "Electrical power Pe (W)"

== system powerlib/Machines/Simplified Synchronous Machine pu Units/Measurement list ==
  In1 : Inport  Port=1  LatchInput=off
  Bus Creator1 : BusCreator  DialogController=Simulink.DDGSource_Bus  Inputs=12
  Demux : Demux  Outputs=[1,1,1,1,1,1,1,1,1,1,1,1]
  Out1 : Outport
  wires:
  Demux/12 -> Bus Creator1/12  "Electrical power Pe (pu)"
  Demux/11 -> Bus Creator1/11  "Rotor speed wm (pu)"
  Demux/10 -> Bus Creator1/10  "Rotor angle theta (rad)"
  Demux/9 -> Bus Creator1/9  "Internal voltage Ec (pu)"
  Demux/8 -> Bus Creator1/8  "Internal voltage Eb (pu)"
  Demux/7 -> Bus Creator1/7  "Internal voltage Ea (pu)"
  Demux/6 -> Bus Creator1/6  "Terminal voltage Vc (pu)"
  Demux/5 -> Bus Creator1/5  "Terminal voltage Vb (pu)"
  Demux/4 -> Bus Creator1/4  "Terminal voltage Va (pu)"
  Demux/3 -> Bus Creator1/3  "Stator current is_c (pu)"
  Demux/2 -> Bus Creator1/2  "Stator current is_b (pu)"
  Demux/1 -> Bus Creator1/1  "Stator current is_a (pu)"
  Bus Creator1/1 -> Out1/1
  In1/1 -> Demux/1

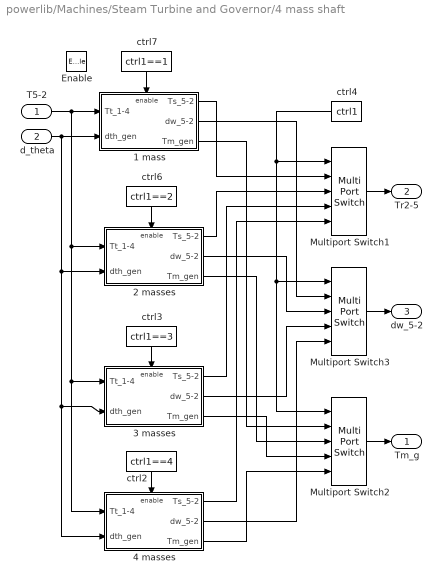
== system powerlib/Machines/Steam Turbine and Governor/4 mass shaft ==
  T5-2 : Inport  Port=1  LatchInput=off
  d_theta : Inport  Port=2  LatchInput=off
  Enable : EnablePort
  1 mass : Subsystem  TreatAsAtomicUnit=on
  2 masses : Subsystem  TreatAsAtomicUnit=on
  3 masses : Subsystem  TreatAsAtomicUnit=on
  4 masses : Subsystem  TreatAsAtomicUnit=on
  Multiport Switch1 : MultiPortSwitch  InputSameDT=on
  Multiport Switch2 : MultiPortSwitch  InputSameDT=on
  Multiport Switch3 : MultiPortSwitch  InputSameDT=on
  ctrl2 : Constant  Orientation=down  Value=ctrl1==4
  ctrl3 : Constant  Orientation=down  Value=ctrl1==3
  ctrl4 : Constant  Orientation=left  Value=ctrl1
  ctrl6 : Constant  Orientation=down  Value=ctrl1==2
  ctrl7 : Constant  Orientation=down  Value=ctrl1==1
  Tm_g : Outport  OutputWhenDisabled=reset  InitialOutput=0
  Tr2-5 : Outport  Port=2  OutputWhenDisabled=reset  InitialOutput=[0 0 0 0]
  dw_5-2 : Outport  Port=3  OutputWhenDisabled=reset  InitialOutput=[0 0 0 0]
  wires:
  1 mass/1(Ts_5-2) -> Multiport Switch1/2
  2 masses/1(Ts_5-2) -> Multiport Switch1/3
  3 masses/1(Ts_5-2) -> Multiport Switch1/4
  4 masses/1(Ts_5-2) -> Multiport Switch1/5
  T5-2/1 -> 1 mass/1(Tt_1-4), 2 masses/1(Tt_1-4), 3 masses/1(Tt_1-4), 4 masses/1(Tt_1-4)
  d_theta/1 -> 1 mass/2(dth_gen), 2 masses/2(dth_gen), 3 masses/2(dth_gen), 4 masses/2(dth_gen)
  1 mass/3(Tm_gen) -> Multiport Switch2/2
  ctrl4/1 -> Multiport Switch1/1, Multiport Switch2/1, Multiport Switch3/1
  2 masses/3(Tm_gen) -> Multiport Switch2/3
  3 masses/3(Tm_gen) -> Multiport Switch2/4
  4 masses/3(Tm_gen) -> Multiport Switch2/5
  ctrl2/1 -> 4 masses/Enable
  ctrl3/1 -> 3 masses/Enable
  1 mass/2(dw_5-2) -> Multiport Switch3/2
  2 masses/2(dw_5-2) -> Multiport Switch3/3
  ctrl7/1 -> 1 mass/Enable
  ctrl6/1 -> 2 masses/Enable
  3 masses/2(dw_5-2) -> Multiport Switch3/4
  Multiport Switch1/1 -> Tr2-5/1
  Multiport Switch2/1 -> Tm_g/1
  Multiport Switch3/1 -> dw_5-2/1
  4 masses/2(dw_5-2) -> Multiport Switch3/5

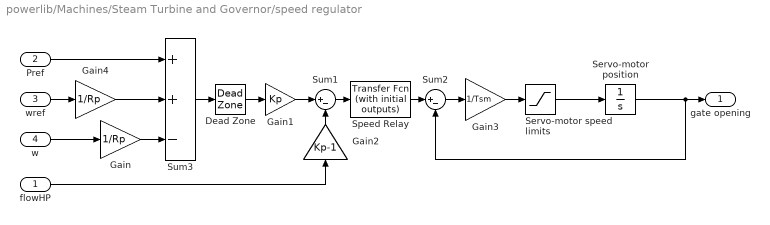
== system powerlib/Machines/Steam Turbine and Governor/speed regulator ==
  flowHP : Inport  Port=1  LatchInput=off
  Pref : Inport  Port=2  LatchInput=off
  wref : Inport  Port=3  LatchInput=off
  w : Inport  Port=4  LatchInput=off
  Dead Zone : DeadZone  LowerValue=-Dz  UpperValue=Dz  SaturateOnIntegerOverflow=on
  Gain : Gain  Gain=1/Rp  SaturateOnIntegerOverflow=on
  Gain1 : Gain  Gain=Kp  SaturateOnIntegerOverflow=on
  Gain2 : Gain  Orientation=up  Gain=Kp-1  SaturateOnIntegerOverflow=on
  Gain3 : Gain  Gain=1/Tsm  SaturateOnIntegerOverflow=on
  Gain4 : Gain  Gain=1/Rp  SaturateOnIntegerOverflow=on
  Servo-motor position : Integrator  InitialCondition=g0  LimitOutput=on  UpperSaturationLimit=gmax  LowerSaturationLimit=gmin
  Servo-motor speed limits : Saturate  UpperLimit=vgmax  LowerLimit=vgmin
  Speed Relay : simulink_extras/Additional Linear/Transfer Fcn (with initial outputs)  N=[1]  D=[Tsr 1]  Y0=g0  U0=g0
  Sum1 : Sum  Inputs=|+-  SaturateOnIntegerOverflow=on  InputSameDT=on
  Sum2 : Sum  Inputs=|+-  SaturateOnIntegerOverflow=on  InputSameDT=on
  Sum3 : Sum  Inputs=++-  SaturateOnIntegerOverflow=on  InputSameDT=on
  gate opening : Outport
  wires:
  Servo-motor speed limits/1 -> Servo-motor position/1
  Gain3/1 -> Servo-motor speed limits/1
  Sum2/1 -> Gain3/1
  Speed Relay/1 -> Sum2/1
  Sum1/1 -> Speed Relay/1
  Gain2/1 -> Sum1/2
  Gain1/1 -> Sum1/1
  Dead Zone/1 -> Gain1/1
  wref/1 -> Gain4/1
  Sum3/1 -> Dead Zone/1
  w/1 -> Gain/1
  Gain/1 -> Sum3/3
  Pref/1 -> Sum3/1
  Gain4/1 -> Sum3/2
  flowHP/1 -> Gain2/1
  Servo-motor position/1 -> gate opening/1, Sum2/2

== system powerlib/Machines/Steam Turbine and Governor/steam turbine ==
  gate : Inport  Port=1  LatchInput=off
  Pboil : Inport  Port=2  LatchInput=off
  Gain : Gain  Gain=F2  SaturateOnIntegerOverflow=on
  Gain2 : Gain  Gain=F3  SaturateOnIntegerOverflow=on
  Gain3 : Gain  Gain=F4  SaturateOnIntegerOverflow=on
  Gain4 : Gain  Gain=F5  SaturateOnIntegerOverflow=on
  Mux : Mux
  Product : Product  SaturateOnIntegerOverflow=on  InputSameDT=on
  Stage1 : Subsystem
  Stage2 : Subsystem
  "Stage3 " : Subsystem
  Stage4 : Subsystem
  flowHp : Outport
  T5-2 : Outport  Port=2
  wires:
  Mux/1 -> T5-2/1
  Stage4/1(Out1) -> Gain/1
  "Stage3 "/1(Out1) -> Stage4/1(In1), Gain2/1
  Gain/1 -> Mux/4
  Gain2/1 -> Mux/3
  Gain3/1 -> Mux/2
  Gain4/1 -> Mux/1
  Stage2/1(Out1) -> "Stage3 "/1(In1), Gain3/1
  Product/1 -> Stage1/1(In1)
  Stage1/1(Out1) -> flowHp/1, Stage2/1(In1), Gain4/1
  gate/1 -> Product/1
  Pboil/1 -> Product/2

== system powerlib/Machines/Synchronous Machine SI Fundamental/Measurement list ==
  m_e : Inport  Port=1  LatchInput=off
  m_m : Inport  Port=2  LatchInput=off
  Bus Creator1 : BusCreator  DialogController=Simulink.DDGSource_Bus  Inputs="'Stator current','dq0 components','Mechanical','Load angle   delta  (deg)','Output active power   Peo (W)','Output reactive power  Qeo (W)'"
  Bus Creator2 : BusCreator  DialogController=Simulink.DDGSource_Bus  Inputs=3
  Bus Creator3 : BusCreator  DialogController=Simulink.DDGSource_Bus  Inputs=10
  Bus Creator4 : BusCreator  DialogController=Simulink.DDGSource_Bus  Inputs=6
  Demux : Demux  Outputs=[1,1,1,1,1,1,1,1,1,1,1,1,1,1,1,1]
  Demux1 : Demux  Outputs=[1,1,1,1,1,1]
  m : Outport
  wires:
  Bus Creator4/1 -> Bus Creator1/3  "Mechanical"
  Bus Creator3/1 -> Bus Creator1/2  "dq0 components"
  Demux/13 -> Bus Creator3/10  "Stator voltage  vd (V)"
  Demux/12 -> Bus Creator3/9  "Stator voltage  vq (V)"
  Demux/11 -> Bus Creator3/8  "Mutual flux  phimd (V s)"
  Demux/10 -> Bus Creator3/7  "Mutual flux  phimq (V s)"
  Demux/9 -> Bus Creator3/6  "Damper winding current  ikd (A)"
  Demux/8 -> Bus Creator3/5  "Damper winding current  ikq2 (A)"
  Demux/7 -> Bus Creator3/4  "Damper winding current  ikq1 (A)"
  Demux/6 -> Bus Creator3/3  "Field current  ifd (A)"
  Demux/5 -> Bus Creator3/2  "Stator current  id (A)"
  Demux/4 -> Bus Creator3/1  "Stator current  iq (A)"
  Bus Creator2/1 -> Bus Creator1/1  "Stator current"
  Demux/3 -> Bus Creator2/3  "is_c (A)"
  Demux/2 -> Bus Creator2/2  "is_b (A)"
  Demux/1 -> Bus Creator2/1  "is_a (A)"
  Bus Creator1/1 -> m/1
  m_e/1 -> Demux/1
  m_m/1 -> Demux1/1
  Demux1/1 -> Bus Creator4/1  "Rotor angle deviation  d_theta (rad)"
  Demux1/2 -> Bus Creator4/2  "Rotor speed  wm (rad/s)"
  Demux1/3 -> Bus Creator4/3  "Electrical power  Pe (W)"
  Demux1/4 -> Bus Creator4/4  "Rotor speed deviation  dw (pu)"
  Demux1/5 -> Bus Creator4/5  "Rotor mechanical angle  theta (deg)"
  Demux1/6 -> Bus Creator4/6  "Electromagnetic torque  Te (N*m)"
  Demux/14 -> Bus Creator1/4  "Load angle   delta  (deg)"
  Demux/15 -> Bus Creator1/5  "Output active power   Peo (W)"
  Demux/16 -> Bus Creator1/6  "Output reactive power  Qeo (W)"

== system powerlib/Machines/Synchronous Machine pu Fundamental/Measurement list ==
  m_e : Inport  Port=1  LatchInput=off
  m_m : Inport  Port=2  LatchInput=off
  Bus Creator1 : BusCreator  DialogController=Simulink.DDGSource_Bus  Inputs="'Stator current','dq0 components','Mechanical','Load angle   delta  (deg)','Output active power   Peo (pu)','Output reactive power  Qeo (pu)'"
  Bus Creator2 : BusCreator  DialogController=Simulink.DDGSource_Bus  Inputs=3
  Bus Creator3 : BusCreator  DialogController=Simulink.DDGSource_Bus  Inputs=10
  Bus Creator4 : BusCreator  DialogController=Simulink.DDGSource_Bus  Inputs=6
  Demux : Demux  Outputs=[1,1,1,1,1,1,1,1,1,1,1,1,1,1,1,1]
  Demux1 : Demux  Outputs=[1,1,1,1,1,1]
  m : Outport
  wires:
  Bus Creator4/1 -> Bus Creator1/3  "Mechanical"
  Bus Creator3/1 -> Bus Creator1/2  "dq0 components"
  Demux/13 -> Bus Creator3/10  "Stator voltage  vd (pu)"
  Demux/12 -> Bus Creator3/9  "Stator voltage  vq (pu)"
  Demux/11 -> Bus Creator3/8  "Mutual flux  phimd (pu)"
  Demux/10 -> Bus Creator3/7  "Mutual flux  phimq (pu)"
  Demux/9 -> Bus Creator3/6  "Damper winding current  ikd (pu)"
  Demux/8 -> Bus Creator3/5  "Damper winding current  ikq2 (pu)"
  Demux/7 -> Bus Creator3/4  "Damper winding current  ikq1 (pu)"
  Demux/6 -> Bus Creator3/3  "Field current  ifd (pu)"
  Demux/5 -> Bus Creator3/2  "Stator current  id (pu)"
  Demux/4 -> Bus Creator3/1  "Stator current  iq (pu)"
  Bus Creator2/1 -> Bus Creator1/1  "Stator current"
  Demux/3 -> Bus Creator2/3  "is_c (pu)"
  Demux/2 -> Bus Creator2/2  "is_b (pu)"
  Demux/1 -> Bus Creator2/1  "is_a (pu)"
  Bus Creator1/1 -> m/1
  m_e/1 -> Demux/1
  m_m/1 -> Demux1/1
  Demux1/1 -> Bus Creator4/1  "Rotor angle deviation  d_theta (rad)"
  Demux1/2 -> Bus Creator4/2  "Rotor speed  wm (pu)"
  Demux1/3 -> Bus Creator4/3  "Electrical power  Pe (pu)"
  Demux1/4 -> Bus Creator4/4  "Rotor speed deviation  dw (pu)"
  Demux1/5 -> Bus Creator4/5  "Rotor mechanical angle  theta (deg)"
  Demux1/6 -> Bus Creator4/6  "Electromagnetic torque  Te (pu)"
  Demux/14 -> Bus Creator1/4  "Load angle   delta  (deg)"
  Demux/15 -> Bus Creator1/5  "Output active power   Peo (pu)"
  Demux/16 -> Bus Creator1/6  "Output reactive power  Qeo (pu)"

== system powerlib/Machines/Synchronous Machine pu Standard/Measurement list ==
  m_e : Inport  Port=1  LatchInput=off
  m_m : Inport  Port=2  LatchInput=off
  Bus Creator1 : BusCreator  DialogController=Simulink.DDGSource_Bus  Inputs="'Stator current','dq0 components','Mechanical','Load angle   delta  (deg)','Output active power   Peo (pu)','Output reactive power  Qeo (pu)'"
  Bus Creator2 : BusCreator  DialogController=Simulink.DDGSource_Bus  Inputs=3
  Bus Creator3 : BusCreator  DialogController=Simulink.DDGSource_Bus  Inputs=10
  Bus Creator4 : BusCreator  DialogController=Simulink.DDGSource_Bus  Inputs=6
  Demux : Demux  Outputs=[1,1,1,1,1,1,1,1,1,1,1,1,1,1,1,1]
  Demux1 : Demux  Outputs=[1,1,1,1,1,1]
  m : Outport
  wires:
  Demux/16 -> Bus Creator1/6  "Output reactive power  Qeo (pu)"
  Demux/15 -> Bus Creator1/5  "Output active power   Peo (pu)"
  Demux/14 -> Bus Creator1/4  "Load angle   delta  (deg)"
  Demux1/6 -> Bus Creator4/6  "Electromagnetic torque  Te (pu)"
  Demux1/5 -> Bus Creator4/5  "Rotor mechanical angle  theta (deg)"
  Demux1/4 -> Bus Creator4/4  "Rotor speed deviation  dw (pu)"
  Demux1/3 -> Bus Creator4/3  "Electrical power  Pe (pu)"
  Demux1/2 -> Bus Creator4/2  "Rotor speed  wm  (pu)"
  Demux1/1 -> Bus Creator4/1  "Rotor angle deviation  d_theta (rad)"
  m_m/1 -> Demux1/1
  m_e/1 -> Demux/1
  Bus Creator1/1 -> m/1
  Demux/1 -> Bus Creator2/1  "is_a (pu)"
  Demux/2 -> Bus Creator2/2  "is_b (pu)"
  Demux/3 -> Bus Creator2/3  "is_c (pu)"
  Bus Creator2/1 -> Bus Creator1/1  "Stator current"
  Demux/4 -> Bus Creator3/1  "Stator current  iq (pu)"
  Demux/5 -> Bus Creator3/2  "Stator current  id (pu)"
  Demux/6 -> Bus Creator3/3  "Field current  ifd (pu)"
  Demux/7 -> Bus Creator3/4  "Damper winding current  ikq1 (pu)"
  Demux/8 -> Bus Creator3/5  "Damper winding current  ikq2 (pu)"
  Demux/9 -> Bus Creator3/6  "Damper winding current  ikd (pu)"
  Demux/10 -> Bus Creator3/7  "Mutual flux  phimq (pu)"
  Demux/11 -> Bus Creator3/8  "Mutual flux  phimd (pu)"
  Demux/12 -> Bus Creator3/9  "Stator voltage  vq (pu)"
  Demux/13 -> Bus Creator3/10  "Stator voltage  vd (pu)"
  Bus Creator3/1 -> Bus Creator1/2  "dq0 components"
  Bus Creator4/1 -> Bus Creator1/3  "Mechanical"

== system powerlib/Measurements/Multimeter/StoreData ==
  In1 : Inport  Port=1  LatchInput=off
  Enable : EnablePort  ZeroCross=off
  To Workspace : ToWorkspace  VariableName=LibraryTag  SampleTime=-1  SaveFormat=Structure With Time
  wires:
  In1/1 -> To Workspace/1

== system powerlib/Measurements/Three-Phase V-I Measurement/Ia ==
  Out1 : Outport
  wires:
  [LibraryTag] -> Out1/1

== system powerlib/Measurements/Three-Phase V-I Measurement/Ib ==
  Out1 : Outport
  wires:
  [LibraryTag] -> Out1/1

== system powerlib/Measurements/Three-Phase V-I Measurement/Ic ==
  Out1 : Outport
  wires:
  [LibraryTag] -> Out1/1

== system powerlib/Measurements/Three-Phase V-I Measurement/Vb ==
  Out1 : Outport
  wires:
  [LibraryTag] -> Out1/1

== system powerlib/Measurements/Three-Phase V-I Measurement/Vc ==
  Out1 : Outport
  wires:
  [LibraryTag] -> Out1/1

== system powerlib/Phasor Elements/Static Var Compensator/I1 I2-->Phasors ==
  I1 : Inport  Port=1  LatchInput=off
  I2 : Inport  Port=2  LatchInput=off
  Mux1 : Mux  Inputs=2
  Sum1 : Sum  SaturateOnIntegerOverflow=on  InputSameDT=on
  Sum3 : Sum  SaturateOnIntegerOverflow=on  InputSameDT=on
  a : Gain  Gain=exp(j*2*pi/3)  SaturateOnIntegerOverflow=on
  a^2 : Gain  Gain=exp(-j*2*pi/3)  SaturateOnIntegerOverflow=on
  Ia Ib cmplx : Outport
  wires:
  Mux1/1 -> Ia Ib cmplx/1  "ia ib"
  Sum1/1 -> Mux1/2
  Sum3/1 -> Mux1/1
  a/1 -> Sum1/2
  a^2/1 -> Sum1/1
  I2/1 -> Sum3/2, a/1
  I1/1 -> Sum3/1, a^2/1
